simulink model "path_follow"  (R2023b)
settings: Solver=VariableStepAuto  StartTime=0.0  StopTime=50  FixedStep=0.001  RelTol=1e-3
settings Model: Creator=henry  LastModifiedBy=henry
settings SolverCC: ZeroCrossAlgorithm=Adaptive
settings DebuggingCC: MaskedZcDiagnostic=none  IgnoredZcDiagnostic=none

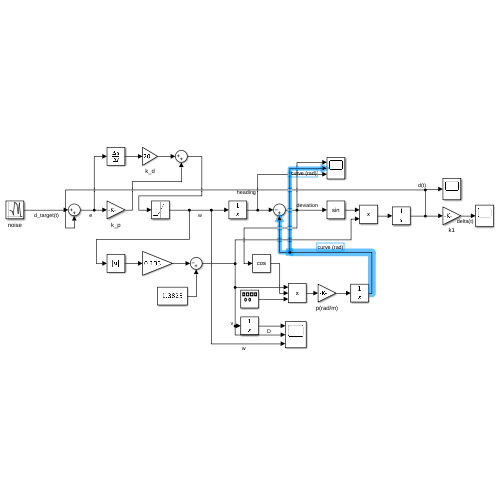
[thumbnail: Simulink's stored preview of the top-level diagram]
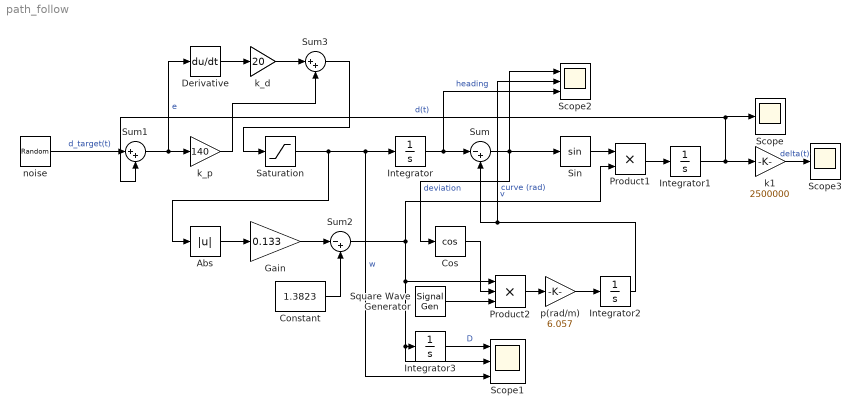
== system path_follow ==
  Abs : Abs  SaturateOnIntegerOverflow=off
  Constant : Constant  Value=1.3823
  Cos : Trigonometry  Operator=cos
  Derivative : Derivative
  Gain : Gain  Gain=0.133
  Integrator{,1..3} (4 alike) : Integrator
  Product1 : Product
  Product2 : Product  Inputs=3
  Saturation : Saturate  UpperLimit=10.3932  LowerLimit=-10.3932
  Scope : Scope
  Scope1 : Scope  NumInputPorts=3
  Scope2 : Scope  NumInputPorts=3
  Scope3 : Scope
  Sin : Trigonometry
  Square Wave Generator : SignalGenerator  WaveForm=square  Frequency=1/10
  Sum : Sum  Inputs=|-+
  Sum1 : Sum  Inputs=|++
  Sum2 : Sum  Inputs=|-+
  Sum3 : Sum  Inputs=|++
  k1 : Gain  Gain=2500000
  k_d : Gain  Gain=20
  k_p : Gain  Gain=140
  "noise " : RandomNumber  Variance=0.001  SampleTime=0.001
  p(rad/m) : Gain  Gain=6.057
  wires:
  "noise "/1 -> Sum1/1  "d_target(t)"
  Abs/1 -> Gain/1
  Gain/1 -> Sum2/1
  Integrator/1 -> Scope2/3, Sum/1  "heading"
  Integrator1/1 -> Scope/1, Sum1/2, k1/1  "d(t)"
  Saturation/1 -> Integrator/1, Scope1/3, Abs/1  "w"
  Constant/1 -> Sum2/2
  Sum2/1 -> Integrator3/1, Scope1/2, Product2/1, Product1/2  "v"
  Sum1/1 -> Derivative/1, k_p/1  "e"
  Sum/1 -> Cos/1, Scope2/1, Sin/1  "deviation"
  Sin/1 -> Product1/1
  Product1/1 -> Integrator1/1
  Integrator2/1 -> Scope2/2, Sum/2  "curve (rad)"
  Product2/1 -> p(rad/m)/1
  p(rad/m)/1 -> Integrator2/1
  Square Wave Generator/1 -> Product2/3
  Integrator3/1 -> Scope1/1  "D"
  Cos/1 -> Product2/2
  Sum3/1 -> Saturation/1
  k_d/1 -> Sum3/1
  k_p/1 -> Sum3/2
  Derivative/1 -> k_d/1
  k1/1 -> Scope3/1  "delta(t)"
